simulink model "motor_PVT_Test"  (R2021b)
settings: Solver=FixedStepAuto  StartTime=0.0  StopTime=300  FixedStep=0.005  RelTol=1e-3  EnableMultiTasking=on
libraries: raspberrypiCommlib x5
settings Model: Creator=The MathWorks, Inc.  LastModifiedBy=kboxi
settings SolverCC: AlgebraicLoopSolver=TrustRegion  PositivePriorityOrder=on
settings OptimizationCC: EnhancedBackFolding=on  PassReuseOutputArgsThreshold=0  MaxStackSize=64  OptimizeBlockOrder=speed  DifferentSizesBufferReuse=on  OptimizationCustomize=off
settings DebuggingCC: ParameterTunabilityLossMsg=error  SFMachineParentedDataDiag=warning
settings HardwareCC: ProdBitPerPointer=32  ProdBitPerSizeT=32  ProdBitPerPtrDiffT=32  ProdLargestAtomicInteger=Long  ProdLargestAtomicFloat=Double  ProdWordSize=32  ProdLongLongMode=on  ProdHWDeviceType=ARM Compatible->ARM Cortex  UseEmbeddedCoderFeatures=off
settings RTWCC: Description=Embedded Coder  SystemTargetFile=ert.tlc  HardwareBoard=Raspberry Pi  TLCOptions="-aInlineSetEventsForThisBaseRateFcn=TLC_FALSE -aSuppressMultiTaskScheduler=TLC_FALSE  -aRateBasedStepFcn=0"  TemplateMakefile=ert_default_tmf  Toolchain=GNU GCC Embedded Linux  BuildConfiguration=Faster Runs
settings CodeAppCC: ForceParamTrailComments=on  OperatorAnnotations=on
settings ERTTargetCC: ERTCustomFileBanners=off  SupportContinuousTime=on  SupportNonInlinedSFcns=on  RemoveResetFunc=off  SupportVariableSizeSignals=on  ModelStepFunctionPrototypeControlCompliant=off  ExtModeTransport=2  ExtModeStaticAlloc=on  ExtModeMexFile=ext_xcp  ExtModeIntrfLevel=Level2 - Open

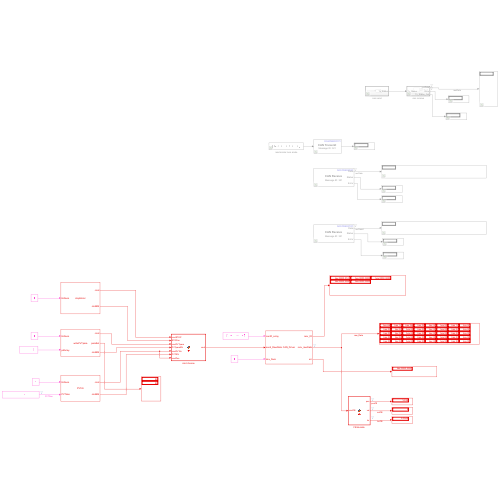
[thumbnail: Simulink's stored preview of the top-level diagram]
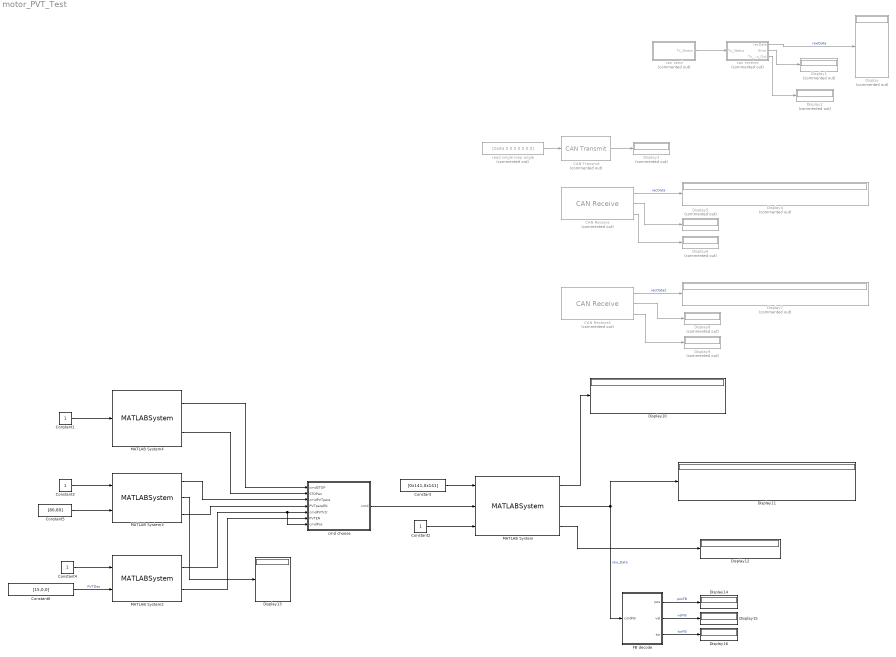
== system motor_PVT_Test ==
  CAN Receive : raspberrypiCommlib/CAN Receive  Commented=on  DeviceID=can1  SetupCAN=off  TypeofCAN=Real  OutputDataType=Raw data  IdentifierType=Standard (11-bit identifier)  MessageId=0x141  MsgLength=8  SampleTime=-1  OutputError=on  OutputRemote=off  SimulateUsing=Code generation
      settings: SourceProductBaseCode=RASPPI
  CAN Receive1 : raspberrypiCommlib/CAN Receive  Commented=on  DeviceID=can0  SetupCAN=off  TypeofCAN=Real  OutputDataType=Raw data  IdentifierType=Standard (11-bit identifier)  MessageId=0x141  MsgLength=8  SampleTime=-1  OutputError=on  OutputRemote=off  SimulateUsing=Code generation
      settings: SourceProductBaseCode=RASPPI
  CAN Transmit : raspberrypiCommlib/CAN Transmit  Commented=on  DeviceID=can1  SetupCAN=off  TypeofCAN=Real  InputDataType=Raw data  BlockingMode_=off  BlockTimeout_=1  OutputStatus=on  IdentifierType=Standard (11-bit identifier)  MessageId=0x141  MsgLength=8  RemoteFrame=off  SimulateUsing=Code generation
      settings: SourceProductBaseCode=RASPPI
  Constant : Constant  Value=[0x141,0x141]  OutDataTypeStr=int32
  Constant1 : Constant
  Constant2 : Constant  OutDataTypeStr=int32
  Constant3 : Constant
  Constant4 : Constant
  Constant5 : Constant  Value=[80,80]
  Constant6 : Constant  Value=[15,0,0]
  Display{,1..9} (10 alike) : Display  Commented=on
      Display settings: Format=hex (Stored Integer)
      Display4 settings: Format=hex (Stored Integer)
      Display7 settings: Format=hex (Stored Integer)
  Display{10..16} (7 alike) : Display
      Display10 settings: Format=hex (Stored Integer)
      Display11 settings: Format=hex (Stored Integer)
      Display12 settings: Format=hex (Stored Integer)
  FB decode : MATLAB Function  TreatAsAtomicUnit=on
  MATLAB System : MATLABSystem  System=canSendRecv  canPort=can1
      mask Type: canSendRecv
      mask Display:
      | disp('CAN_Driver');
      | port_label('input',1,'canID_array');
      | port_label('input',2,'send_RawData');
      | port_label('input',3,'dev_Num');
      | port_label('output',1,'recv_ID');
      | port_label('output',2,'recv_rawData');
      | port_label('output',3,'err');
  MATLAB System2 : MATLABSystem  System=PVTctr  SimulateUsing=Code generation
      mask Type: PVTctr
      mask Display:
      | disp('PVTctr');
      | port_label('input',1,'EnNum');
      | port_label('input',2,'PVTdes');
      | port_label('output',1,'cmd');
      | port_label('output',2,'cmdEN');
  MATLAB System3 : MATLABSystem  System=writePVTpara  SimulateUsing=Code generation
      mask Type: writePVTpara
      mask Display:
      | disp('writePVTpara');
      | port_label('input',1,'EnNum');
      | port_label('input',2,'pdArray');
      | port_label('output',1,'cmd');
      | port_label('output',2,'paraSet');
      | port_label('output',3,'cmdEN');
  MATLAB System4 : MATLABSystem  System=stopMotor  SimulateUsing=Code generation
      mask Type: stopMotor
      mask Display:
      | disp('stopMotor');
      | port_label('input',1,'EnNum');
      | port_label('output',1,'cmd');
      | port_label('output',2,'cmdEN');
  can receive : Subsystem  Commented=on  TreatAsAtomicUnit=on
  can send : Subsystem  Commented=on  TreatAsAtomicUnit=on
  cmd choose : MATLAB Function  TreatAsAtomicUnit=on
  read single loop angle : Constant  Commented=on  Value=[0x94 0 0 0 0 0 0 0]  OutDataTypeStr=uint8
  wires:
  can receive/1(recData) -> Display/1  "rawData"
  can receive/2(Error) -> Display1/1
  can send/1(Tx_Status) -> can receive/1(Tx_Status)
  can receive/3(Tx_Status_Out) -> Display2/1
  read single loop angle/1 -> CAN Transmit/1
  CAN Transmit/1 -> Display3/1
  CAN Receive/1 -> Display4/1  "recData"
  CAN Receive/2 -> Display5/1
  CAN Receive/3 -> Display6/1
  CAN Receive1/1 -> Display7/1  "recData2"
  CAN Receive1/2 -> Display8/1
  CAN Receive1/3 -> Display9/1
  Constant/1 -> MATLAB System/1
  Constant2/1 -> MATLAB System/3
  MATLAB System/1 -> Display10/1
  MATLAB System/2 -> Display11/1, FB decode/1(cmdFB)  "raw_Data"
  MATLAB System/3 -> Display12/1
  Constant1/1 -> MATLAB System4/1
  Constant3/1 -> MATLAB System3/1
  Constant4/1 -> MATLAB System2/1
  cmd choose/1(cmd) -> MATLAB System/2
  MATLAB System4/1 -> cmd choose/1(cmdSTOP)
  MATLAB System4/2 -> cmd choose/2(STOPen)
  MATLAB System3/1 -> cmd choose/3(cmdPVTpara)
  MATLAB System3/3 -> cmd choose/4(PVTparaEN)
  MATLAB System2/1 -> cmd choose/5(cmdPVTctr), cmd choose/7(cmdPos)
  MATLAB System2/2 -> cmd choose/6(PVTEN)
  Constant5/1 -> MATLAB System3/2
  Constant6/1 -> MATLAB System2/2  "PVTDes"
  MATLAB System3/2 -> Display13/1
  FB decode/1(pos) -> Display14/1  "posFB"
  FB decode/2(vel) -> Display15/1  "velFB"
  FB decode/3(tor) -> Display16/1  "torFB"

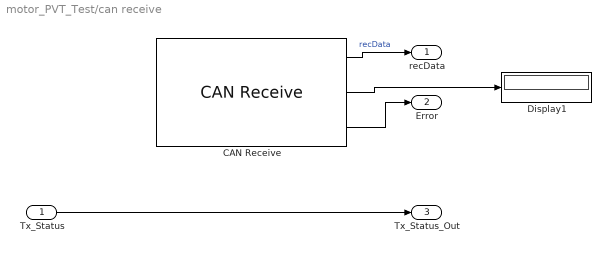
== system motor_PVT_Test/can receive ==
  Tx_Status : Inport
  CAN Receive : raspberrypiCommlib/CAN Receive  DeviceID=can1  SetupCAN=on  TypeofCAN=Real  OutputDataType=Raw data  IdentifierType=Standard (11-bit identifier)  MessageId=0x141  MsgLength=8  SampleTime=-1  OutputError=on  OutputRemote=off  SimulateUsing=Code generation
      settings: SourceProductBaseCode=RASPPI
  Display1 : Display
  recData : Outport
  Error : Outport  Port=2
  Tx_Status_Out : Outport  Port=3
  wires:
  CAN Receive/1 -> recData/1  "recData"
  CAN Receive/2 -> Display1/1
  CAN Receive/3 -> Error/1
  Tx_Status/1 -> Tx_Status_Out/1

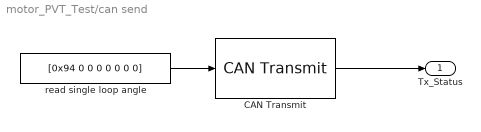
== system motor_PVT_Test/can send ==
  CAN Transmit : raspberrypiCommlib/CAN Transmit  DeviceID=can1  SetupCAN=on  TypeofCAN=Real  InputDataType=Raw data  BlockingMode_=off  BlockTimeout_=1  OutputStatus=on  IdentifierType=Standard (11-bit identifier)  MessageId=0x141  MsgLength=8  RemoteFrame=off  SimulateUsing=Code generation
      settings: SourceProductBaseCode=RASPPI
  read single loop angle : Constant  Value=[0x94 0 0 0 0 0 0 0]  OutDataTypeStr=uint8
  Tx_Status : Outport
  wires:
  read single loop angle/1 -> CAN Transmit/1
  CAN Transmit/1 -> Tx_Status/1

== matlab function motor_PVT_Test/cmd choose ==
  data: cmdSTOP input; cmd output; STOPen input; cmdPVTpara input; PVTparaEN input; cmdPVTctr input; PVTEN input; cmdPos input
function cmd = fcn(cmdSTOP,STOPen,cmdPVTpara,PVTparaEN,cmdPVTctr,PVTEN,cmdPos)
if STOPen>0.5
    cmd=cmdSTOP;
    return;
end
if PVTparaEN>0.5
    cmd=cmdPVTpara;
    return;
end
if PVTEN>0.5
    cmd=cmdPVTctr;
    return;
end
cmd=cmdPos;

== matlab function motor_PVT_Test/FB decode ==
  data: cmdFB input uint8; pos output; vel output; tor output
function [pos,vel,tor] = fcn(cmdFB)
%data=[u(2:8);0x00];
%y = double(typecast(u(7:8),'uint16'))*0.01;
pos = double(typecast(cmdFB(3:4),'int16'))*0.01;
vel = double(typecast(cmdFB(5:6),'int16'));
tor = double(typecast(cmdFB(7:8),'int16'))*66/4096;
